simulink model "Q1_iven"  (R2016b)
settings: Solver=FixedStepAuto  StartTime=0.0  StopTime=.1  FixedStep=0.00001  RelTol=1e-3
libraries: powerlib x10
settings Model: Creator=Gulten  LastModifiedBy=Gulten

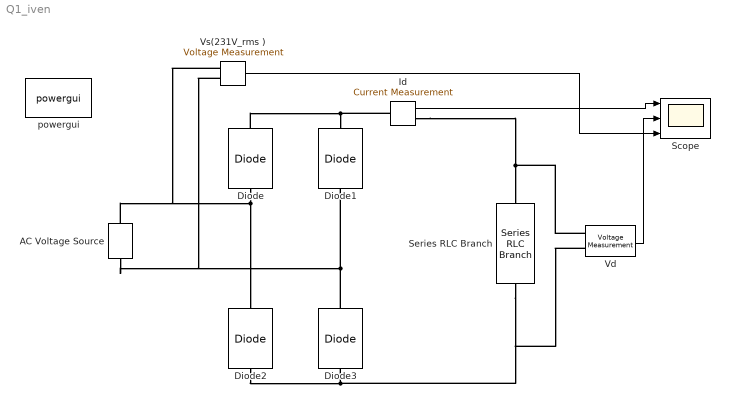
== system Q1_iven ==
  AC Voltage Source : powerlib/Electrical Sources/AC Voltage Source  Amplitude=326.6  Phase=0  Frequency=50  SampleTime=0  Measurements=None  BusType=swing  Pref=10e3  Qref=0  Qmin=-inf  Qmax=+inf
  Diode{,1..3} (4 alike) : powerlib/Power Electronics/Diode  Ron=0  Lon=0  Vf=0  IC=0  UseSnubber=off  Rs=inf  Cs=inf  Measurements=off
  Id : powerlib/Measurements/Current Measurement  PhasorSimulation=off  OutputType=Complex  PSBequivalent=0
  Scope : Scope  NumInputPorts=3
  Series RLC Branch : powerlib/Elements/Series RLC Branch  LConnTagsString=__new0  RConnTagsString=__new0  BranchType=R  Resistance=100  Inductance=1e-3  SetiL0=off  InitialCurrent=0  Capacitance=1e-6  Setx0=off  InitialVoltage=0  Measurements=None
  Vd : powerlib/Measurements/Voltage Measurement  PhasorSimulation=off  OutputType=Complex  PSBequivalent=0
  Vs(231V_rms ) : powerlib/Measurements/Voltage Measurement  PhasorSimulation=off  OutputType=Complex  PSBequivalent=0
  powergui : powerlib/powergui  Priority=1  SimulationMode=Continuous  SolverType=Tustin/Backward Euler (TBE)  SampleTime=50e-6  frequency=60  SPID=on  DisableSnubberDevices=off  DisableRonSwitches=off  DisableVfSwitches=off  SwTol=0  DisplayEquations=off  Interpol=off  ExternalGateDelay=off  methode=off  Ts=10  FunctionMessages=off  echomessages=off  HookPort=off  EnableUseOfTLC=off  x0status=blocks  frequencyindice=50  Pbase=100e6  ErrMax=1e-4  Iterations=50  UnitsV=kV  UnitsW=MW  buscounter=0  RestoreLinks=warning  ResistiveCurrentMeasurement=off  Frange=[0:2:500]  Ylog=off  Xlog=on  ShowGrid=off  save=off  variable=ZData  structure=0  ZoomFFT=off  StartTime=0.0  cycles=1  DisplayStyle=1  fundamental=60  FreqAxis=off  MaxFrequency=1000  frequencyindicesteady=1  RmsSteady=1  display=off
  wires:
  Id/1 -> Scope/1
  Vd/1 -> Scope/2
  Vs(231V_rms )/1 -> Scope/3
  connections:
  Diode/LConn1 -- Vs(231V_rms )/LConn1 -- AC Voltage Source/RConn1 -- Diode2/RConn1
  Diode3/RConn1 -- Vs(231V_rms )/LConn2 -- AC Voltage Source/LConn1 -- Diode1/LConn1
  Diode/RConn1 -- Id/LConn1 -- Diode1/RConn1
  Diode2/LConn1 -- Vd/LConn2 -- Series RLC Branch/LConn1 -- Diode3/LConn1
  Id/RConn1 -- Vd/LConn1 -- Series RLC Branch/RConn1
